simulink model "EEG_Record"  (R2014a)
settings: Solver=FixedStepDiscrete  StartTime=0.0  StopTime=inf  FixedStep=1/256  RelTol=1e-3  EnableMultiTasking=on
InitFcn:
  | set_param('EEG_Record/Subsystem1/Gain1','Gain','0');
  | set_param('EEG_Record/Stop_Simulation','value','0');
  | 
  | ts=1/256;
StartFcn:
  | P300_Panel_Setting
undefined symbols (not defined in the file or in its folder): currentCFG_EEG_Record_UA, UA
libraries: Tools x2, gUSBamplib x1
settings Model: Creator=BIOLABB  LastModifiedBy=BCI1
settings OptimizationCC: BlockReduction=off  BooleanDataType=off  SimCompilerOptimization=off
settings DebuggingCC: SaveWithParameterizedLinksMsg=none  UnderspecifiedInitializationDetection=Classic  SignalResolutionControl=TryResolveAllWithWarning  SolverPrmCheckMsg=none  FcnCallInpInsideContextMsg=error  FrameProcessingCompatibilityMsg=error  SFExecutionAtInitializationDiag=none
settings HardwareCC: ProdBitPerSizeT=32  ProdBitPerPtrDiffT=32  TargetUnknown=on
settings RTWCC: RTWCompilerOptimization=off
settings ConfigComp: CovMetricSettings=dw  CovHtmlReporting=on  CovSaveCumulativeToWorkspaceVar=on  CovSaveSingleToWorkspaceVar=on  CovExternalEMLEnable=off  CovSFcnEnable=off

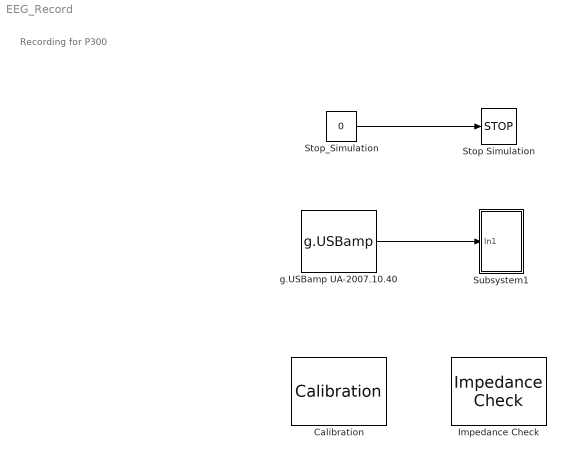
== system EEG_Record ==
  note: Recording for P300
  Calibration : Tools/Calibration  SystemSampleTime=-1
  Impedance Check : Tools/Impedance Check  SystemSampleTime=-1
  Stop Simulation : Stop
  Stop_Simulation : Constant  Value=0  SampleTime=ts
  Subsystem1 : Subsystem
  g.USBamp UA-2007.10.40 : gUSBamplib/g.USBamp  Priority=2  cfg=currentCFG_EEG_Record_UA-2007.10.40.cfg  snr=UA-2007.10.40
  wires:
  g.USBamp UA-2007.10.40/1 -> Subsystem1/1(In1)
  Stop_Simulation/1 -> Stop Simulation/1

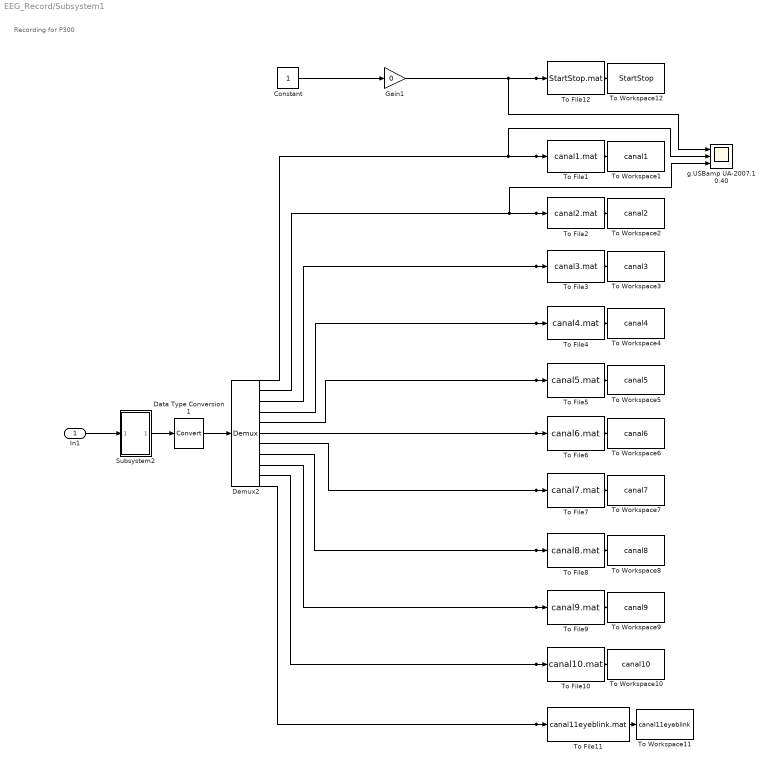
== system EEG_Record/Subsystem1 ==
  note: Recording for P300
  In1 : Inport
  Constant : Constant
  Data Type Conversion1 : DataTypeConversion  SampleTime=ts  SaturateOnIntegerOverflow=on  RndMeth=Zero
  Demux2 : Demux  Outputs=11
  Gain1 : Gain  Gain=0
  Subsystem2 : Subsystem
  To File1 : ToFile  Filename=canal1.mat  MatrixName=canal1  SampleTime=ts
  To File10 : ToFile  Filename=canal10.mat  MatrixName=canal10  SampleTime=ts
  To File11 : ToFile  Filename=canal11eyeblink.mat  MatrixName=canal11eyeblink  SampleTime=ts
  To File12 : ToFile  Filename=StartStop.mat  MatrixName=StartStop  SampleTime=ts
  To File2 : ToFile  Filename=canal2.mat  MatrixName=canal2  SampleTime=ts
  To File3 : ToFile  Filename=canal3.mat  MatrixName=canal3  SampleTime=ts
  To File4 : ToFile  Filename=canal4.mat  MatrixName=canal4  SampleTime=ts
  To File5 : ToFile  Filename=canal5.mat  MatrixName=canal5  SampleTime=ts
  To File6 : ToFile  Filename=canal6.mat  MatrixName=canal6  SampleTime=ts
  To File7 : ToFile  Filename=canal7.mat  MatrixName=canal7  SampleTime=ts
  To File8 : ToFile  Filename=canal8.mat  MatrixName=canal8  SampleTime=ts
  To File9 : ToFile  Filename=canal9.mat  MatrixName=canal9  SampleTime=ts
  To Workspace1 : ToWorkspace  VariableName=canal1  SampleTime=ts
  To Workspace10 : ToWorkspace  VariableName=canal10  SampleTime=ts
  To Workspace11 : ToWorkspace  VariableName=canal11eyeblink  SampleTime=ts
  To Workspace12 : ToWorkspace  VariableName=StartStop  SampleTime=ts
  To Workspace2 : ToWorkspace  VariableName=canal2  SampleTime=ts
  To Workspace3 : ToWorkspace  VariableName=canal3  SampleTime=ts
  To Workspace4 : ToWorkspace  VariableName=canal4  SampleTime=ts
  "To Workspace5 " : ToWorkspace  VariableName=canal5  SampleTime=ts
  "To Workspace6 " : ToWorkspace  VariableName=canal6  SampleTime=ts
  To Workspace7 : ToWorkspace  VariableName=canal7  SampleTime=ts
  To Workspace8 : ToWorkspace  VariableName=canal8  SampleTime=ts
  To Workspace9 : ToWorkspace  VariableName=canal9  SampleTime=ts
  g.USBamp UA-2007.10.40 : Scope  NumInputPorts=3
  wires:
  Subsystem2/1(Out2) -> Data Type Conversion1/1
  In1/1 -> Subsystem2/1(In1)
  Data Type Conversion1/1 -> Demux2/1
  Demux2/11 -> To Workspace11/1, To File11/1
  Demux2/3 -> To Workspace3/1, To File3/1
  Demux2/5 -> "To Workspace5 "/1, To File5/1
  Demux2/7 -> To Workspace7/1, To File7/1
  Demux2/8 -> To Workspace8/1, To File8/1
  Demux2/10 -> To Workspace10/1, To File10/1
  Demux2/4 -> To Workspace4/1, To File4/1
  Demux2/6 -> "To Workspace6 "/1, To File6/1
  Demux2/9 -> To Workspace9/1, To File9/1
  Gain1/1 -> g.USBamp UA-2007.10.40/1, To Workspace12/1, To File12/1
  Demux2/2 -> To Workspace2/1, To File2/1, g.USBamp UA-2007.10.40/3
  Demux2/1 -> To Workspace1/1, To File1/1, g.USBamp UA-2007.10.40/2
  Constant/1 -> Gain1/1

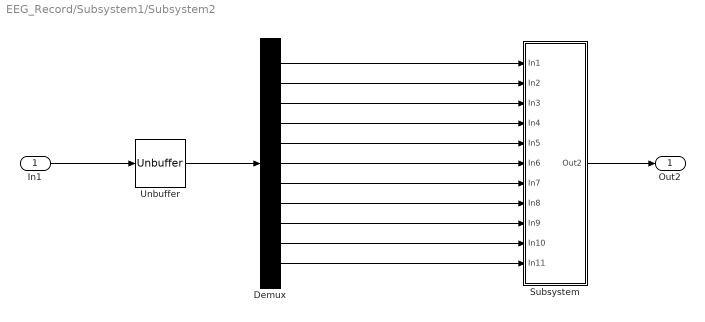
== system EEG_Record/Subsystem1/Subsystem2 ==
  In1 : Inport
  Demux : Demux  Outputs=11
  Subsystem : Subsystem
  Unbuffer : Unbuffer
  Out2 : Outport
  wires:
  Unbuffer/1 -> Demux/1
  In1/1 -> Unbuffer/1
  Subsystem/1(Out2) -> Out2/1
  Demux/1 -> Subsystem/1(In1)
  Demux/2 -> Subsystem/2(In2)
  Demux/3 -> Subsystem/3(In3)
  Demux/4 -> Subsystem/4(In4)
  Demux/5 -> Subsystem/5(In5)
  Demux/6 -> Subsystem/6(In6)
  Demux/7 -> Subsystem/7(In7)
  Demux/8 -> Subsystem/8(In8)
  Demux/9 -> Subsystem/9(In9)
  Demux/10 -> Subsystem/10(In10)
  Demux/11 -> Subsystem/11(In11)

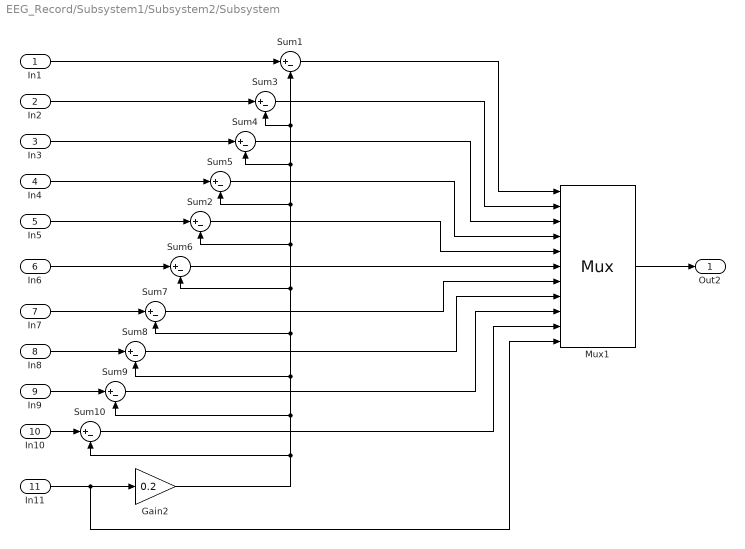
== system EEG_Record/Subsystem1/Subsystem2/Subsystem ==
  In1 : Inport
  In2 : Inport  Port=2
  In3 : Inport  Port=3
  In4 : Inport  Port=4
  In5 : Inport  Port=5
  In6 : Inport  Port=6
  In7 : Inport  Port=7
  In8 : Inport  Port=8
  In9 : Inport  Port=9
  In10 : Inport  Port=10
  In11 : Inport  Port=11
  Gain2 : Gain  Gain=0.2  SampleTime=ts
  Mux1 : Mux  Inputs=11
  Sum{1..10} (10 alike) : Sum  Inputs=|+-  SampleTime=ts
  Out2 : Outport
  wires:
  In11/1 -> Gain2/1, Mux1/11
  In1/1 -> Sum1/1
  In2/1 -> Sum3/1
  In3/1 -> Sum4/1
  In4/1 -> Sum5/1
  Mux1/1 -> Out2/1
  Gain2/1 -> Sum10/2, Sum9/2, Sum8/2, Sum7/2, Sum6/2, Sum2/2, Sum5/2, Sum4/2, Sum3/2, Sum1/2
  In5/1 -> Sum2/1
  In6/1 -> Sum6/1
  In7/1 -> Sum7/1
  In8/1 -> Sum8/1
  In9/1 -> Sum9/1
  In10/1 -> Sum10/1
  Sum1/1 -> Mux1/1
  Sum3/1 -> Mux1/2
  Sum4/1 -> Mux1/3
  Sum5/1 -> Mux1/4
  Sum2/1 -> Mux1/5
  Sum6/1 -> Mux1/6
  Sum7/1 -> Mux1/7
  Sum8/1 -> Mux1/8
  Sum9/1 -> Mux1/9
  Sum10/1 -> Mux1/10
